simulink model "modeloInfeccion3Ejercicio3"  (R2021a)
settings: Solver=VariableStepAuto  StartTime=0.0  StopTime=1000  RelTol=1e-6
undefined symbols (not defined in the file): sigbuilder_block
settings Model: Creator=jmata  LastModifiedBy=jmata

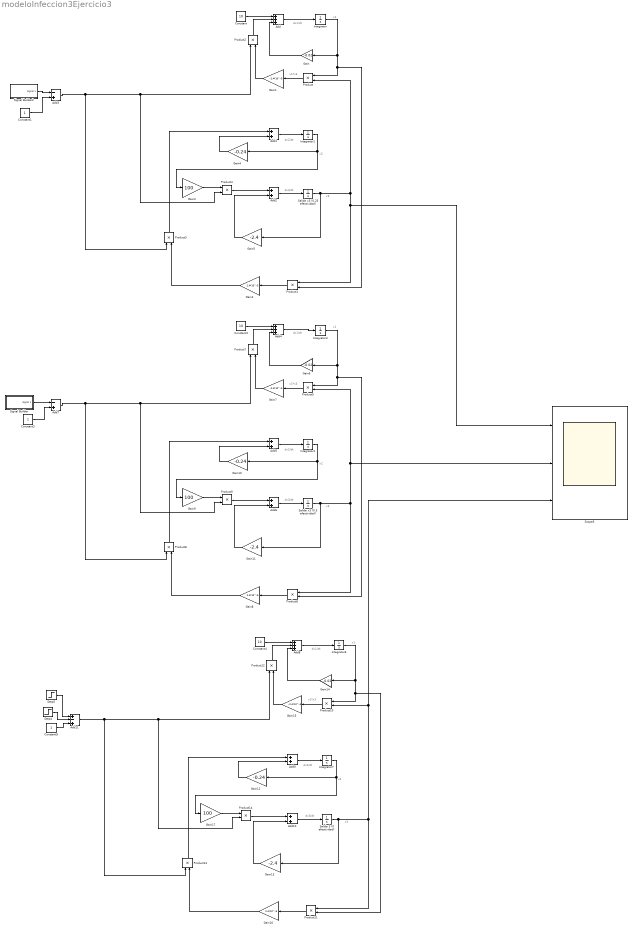
== system modeloInfeccion3Ejercicio3 ==
  note: dx2/dt
  note: dx3/dt
  note: x2
  note: x1*x3
  note: x3
  note: x1
  note: dx1/dt
  note: dx2/dt
  note: dx3/dt
  note: x2
  note: x1*x3
  note: x3
  note: x1
  note: dx1/dt
  note: dx2/dt
  note: dx3/dt
  note: x2
  note: x1*x3
  note: x3
  note: x1
  note: dx1/dt
  Add : Sum  Inputs=+++
  Add{1..2,5..6,9..10} (6 alike) : Sum
  Add11 : Sum  Inputs=+-+
  Add3 : Sum  Inputs=-+
  Add4 : Sum  Inputs=+++
  Add7 : Sum  Inputs=-+
  Add8 : Sum  Inputs=+++
  Constant : Constant  Value=10
  Constant1 : Constant
  Constant2 : Constant  Value=10
  Constant3 : Constant
  Constant4 : Constant  Value=10
  Constant5 : Constant
  Gain : Gain  Gain=-0.02
  Gain1 : Gain  Gain=-2.4*10^-5
  Gain10 : Gain  Gain=-0.24
  Gain11 : Gain  Gain=-2.4
  Gain12 : Gain  Gain=-0.24
  Gain13 : Gain  Gain=-2.4
  Gain14 : Gain  Gain=-0.02
  Gain15 : Gain  Gain=-2.4*10^-5
  Gain16 : Gain  Gain=2.4*10^-5
  Gain17 : Gain  Gain=100
  Gain2 : Gain  Gain=2.4*10^-5
  Gain3 : Gain  Gain=100
  Gain4 : Gain  Gain=-0.24
  Gain5 : Gain  Gain=-2.4
  Gain6 : Gain  Gain=-0.02
  Gain7 : Gain  Gain=-2.4*10^-5
  Gain8 : Gain  Gain=2.4*10^-5
  Gain9 : Gain  Gain=100
  Integrator : Integrator  InitialCondition=600
  Integrator1 : Integrator
  Integrator3 : Integrator  InitialCondition=600
  Integrator4 : Integrator
  Integrator6 : Integrator  InitialCondition=600
  Integrator7 : Integrator
  Product{,1..14} (15 alike) : Product
  Salida 3 (0 efectividad) : Integrator  InitialCondition=1
  Salida x3 (0,5 efectividad) : Integrator  InitialCondition=1
  Salida x3 (0.25 efectividad) : Integrator  InitialCondition=1
  Scope3 : Scope  NumInputPorts=3
  Signal Builder : Subsystem  Tag=STV Subsys  LoadFcn=sigbuilder_block('load');  StartFcn=sigbuilder_block('start');  StopFcn=sigbuilder_block('stop');  ClipboardFcn=sigbuilder_block('clipboard');  mask(Sigbuilder block){tuvar=[0:10]}
      mask help: Simulink:masks:SigbuilderBlock_MD
      mask init:
      | if ~strcmp(get_param(bdroot(gcbh),'SimulationStatus'),'stopped') tuvar = sigbuilder_block('maskInit'); end
      settings: CopyFcn=sigbuilder_block('copy');  DeleteFcn=sigbuilder_block('delete');  ModelCloseFcn=sigbuilder_block('modelClose');  PreSaveFcn=sigbuilder_block('preSave');  PauseFcn=sigbuilder_block('pause');  ContinueFcn=sigbuilder_block('continue');  NameChangeFcn=sigbuilder_block('namechange');  OpenFcn=sigbuilder_block('open',[5.4 30 1141.2 522.6 ]);  CloseFcn=sigbuilder_block('close');
      mask Display: plot(0, 0, 100, 100,[2, 2, 32, 32, 2], [68, 8, 8, 68, 68],[32, 2], [38, 38], [32, 19, 2],[53, 60, 44], [32, 17, 17, 2],[16, 16, 31, 31]);txt = getActiveGroup(gcbh);text(2, 100, txt,'verticalAlignment', 'top');
  Signal Builder2 : Subsystem  Tag=STV Subsys  LoadFcn=sigbuilder_block('load');  StartFcn=sigbuilder_block('start');  StopFcn=sigbuilder_block('stop');  ClipboardFcn=sigbuilder_block('clipboard');  mask(Sigbuilder block){tuvar=[0:10]}
      mask help: Simulink:masks:SigbuilderBlock_MD
      mask init:
      | if ~strcmp(get_param(bdroot(gcbh),'SimulationStatus'),'stopped') tuvar = sigbuilder_block('maskInit'); end
      settings: CopyFcn=sigbuilder_block('copy');  DeleteFcn=sigbuilder_block('delete');  ModelCloseFcn=sigbuilder_block('modelClose');  PreSaveFcn=sigbuilder_block('preSave');  PauseFcn=sigbuilder_block('pause');  ContinueFcn=sigbuilder_block('continue');  NameChangeFcn=sigbuilder_block('namechange');  OpenFcn=sigbuilder_block('open',[5.4 30 1141.2 522.6 ]);  CloseFcn=sigbuilder_block('close');
      mask Display: plot(0, 0, 100, 100,[2, 2, 32, 32, 2], [68, 8, 8, 68, 68],[32, 2], [38, 38], [32, 19, 2],[53, 60, 44], [32, 17, 17, 2],[16, 16, 31, 31]);txt = getActiveGroup(gcbh);text(2, 100, txt,'verticalAlignment', 'top');
  Step4 : Step  After=0  SampleTime=150
  Step5 : Step  After=0  SampleTime=500
  wires:
  Gain5/1 -> Add2/2
  Add/1 -> Integrator/1
  Integrator1/1 -> Gain3/1, Gain4/1
  Salida x3 (0.25 efectividad)/1 -> Gain5/1, Scope3/1, Product1/1, Product/2
  Gain4/1 -> Add1/2
  Add2/1 -> Salida x3 (0.25 efectividad)/1
  Product1/1 -> Gain2/1
  Integrator/1 -> Product/1, Product1/2, Gain/1
  Product/1 -> Gain1/1
  Constant/1 -> Add/1
  Gain/1 -> Add/3
  Add1/1 -> Integrator1/1
  Constant1/1 -> Add3/2
  Product2/1 -> Add/2
  Add3/1 -> Product3/1, Product2/1, Product4/2
  Gain1/1 -> Product2/2
  Gain2/1 -> Product3/2
  Product3/1 -> Add1/1
  Gain3/1 -> Product4/1
  Product4/1 -> Add2/1
  Product9/1 -> Add6/1
  Gain9/1 -> Product9/1
  Product8/1 -> Add5/1
  Gain8/1 -> Product8/2
  Gain7/1 -> Product7/2
  Add7/1 -> Product9/2, Product7/1, Product8/1
  Product7/1 -> Add4/2
  Constant3/1 -> Add7/2
  Add5/1 -> Integrator4/1
  Gain6/1 -> Add4/3
  Constant2/1 -> Add4/1
  Product5/1 -> Gain7/1
  Integrator3/1 -> Gain6/1, Product6/2, Product5/1
  Product6/1 -> Gain8/1
  Add6/1 -> Salida x3 (0,5 efectividad)/1
  Gain10/1 -> Add5/2
  Salida x3 (0,5 efectividad)/1 -> Product5/2, Scope3/2, Product6/1, Gain11/1
  Integrator4/1 -> Gain10/1, Gain9/1
  Add4/1 -> Integrator3/1
  Gain11/1 -> Add6/2
  Gain13/1 -> Add10/2
  Add8/1 -> Integrator6/1
  Integrator7/1 -> Gain17/1, Gain12/1
  Gain12/1 -> Add9/2
  Add10/1 -> Salida 3 (0 efectividad)/1
  Product11/1 -> Gain16/1
  Integrator6/1 -> Product10/1, Product11/2, Gain14/1
  Product10/1 -> Gain15/1
  Constant4/1 -> Add8/1
  Gain14/1 -> Add8/3
  Add9/1 -> Integrator7/1
  Step4/1 -> Add11/2
  Constant5/1 -> Add11/3
  Product12/1 -> Add8/2
  Add11/1 -> Product13/1, Product12/1, Product14/2
  Gain15/1 -> Product12/2
  Gain16/1 -> Product13/2
  Product13/1 -> Add9/1
  Gain17/1 -> Product14/1
  Product14/1 -> Add10/1
  Step5/1 -> Add11/1
  Salida 3 (0 efectividad)/1 -> Gain13/1, Scope3/3, Product10/2, Product11/1
  Signal Builder/1(Signal 1) -> Add7/1
  Signal Builder2/1(Signal 1) -> Add3/1

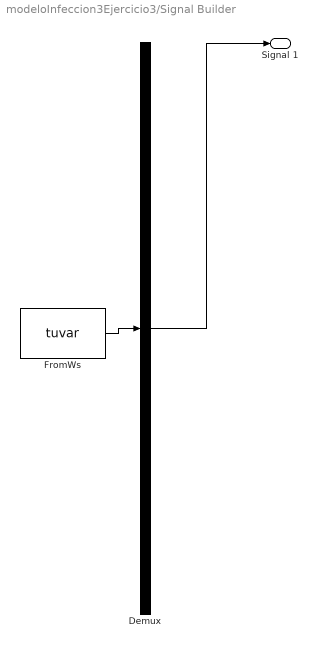
== system modeloInfeccion3Ejercicio3/Signal Builder ==
  Demux : Demux  Tag=STV Demux  Outputs=1
      settings: DisplayOption=none
  FromWs : FromWorkspace  Tag=STV FromWs  VariableName=tuvar
      SigBuilderData=|
      | common.afterFinalStr = 'Extrapolate'
      | common.sampleTime = 0
      | dataSet.timeRange = [0 1000]
      | dataSet.name = 'Group 1'
      | sbobj.Groups.Name = 'Group 1'
      | sbobj.Groups.Signals.Name = 'Signal 1'
      | sbobj.Groups.Signals.XData = [0 150 150 500 500 1000]
      | sbobj.Groups.Signals.YData = [0 0 0.5 0.5 0 -0.005]
      | sbobj.Groups.TimeRange = [0 1000]
  Signal 1 : Outport  Tag=STV Outport
  wires:
  Demux/1 -> Signal 1/1
  FromWs/1 -> Demux/1

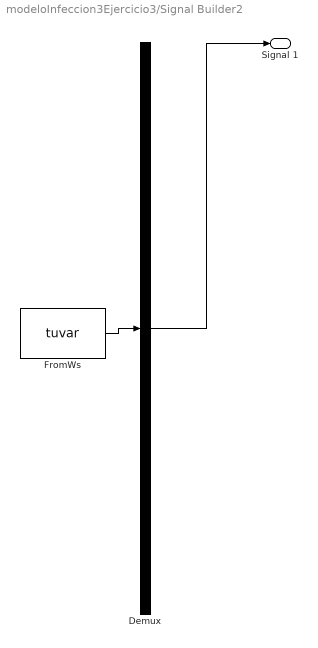
== system modeloInfeccion3Ejercicio3/Signal Builder2 ==
  Demux : Demux  Tag=STV Demux  Outputs=1
      settings: DisplayOption=none
  FromWs : FromWorkspace  Tag=STV FromWs  VariableName=tuvar
      SigBuilderData=|
      | common.afterFinalStr = 'Extrapolate'
      | common.sampleTime = 0
      | dataSet.timeRange = [0 1000]
      | dataSet.name = 'Group 1'
      | sbobj.Groups.Name = 'Group 1'
      | sbobj.Groups.Signals.Name = 'Signal 1'
      | sbobj.Groups.Signals.XData = [0 150 150 500 500 1000]
      | sbobj.Groups.Signals.YData = [0 0 0.25 0.25 0 -0.005]
      | sbobj.Groups.TimeRange = [0 1000]
  Signal 1 : Outport  Tag=STV Outport
  wires:
  Demux/1 -> Signal 1/1
  FromWs/1 -> Demux/1
